simulink model "sfcndemo_stvmgain"  (Simulink 7.6)
settings: Solver=FixedStepDiscrete  SolverMode=SingleTasking  StartTime=0.0  StopTime=4.0  FixedStep=.01  RelTol=1e-3
Description:
  | Time-Varying Matrix Gain C-MEX S-function
settings Model: Creator=The MathWorks Inc.  ExtModeTrigMode=oneshot  ExtModeArmWhenConnect=off  ExtModeAutoUpdateStatusClock=off
settings DataIOCC: LimitDataPoints=off  SaveState=on
settings OptimizationCC: BlockReduction=off  BooleanDataType=off  InitFltsAndDblsToZero=on
settings DebuggingCC: SaveWithParameterizedLinksMsg=none  SignalResolutionControl=TryResolveAllWithWarning  SolverPrmCheckMsg=none  MultiTaskDSMMsg=warning  MultiTaskCondExecSysMsg=none
settings HardwareCC: TargetUnknown=on
settings RTWCC: IncludeERTFirstTime=on
settings CodeAppCC: CustomSymbolStrFcn=$F$N$M
settings GRTTargetCC: TargetFcnLib=ansi_tfl_tmw.mat

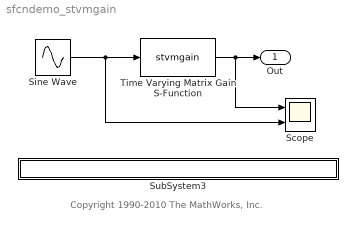
== system sfcndemo_stvmgain ==
  note: Copyright 1990-2010 The MathWorks, Inc.
  Scope : Scope  NumInputPorts=2
      settings: TimeRange=4  YMin=0~-10  YMax=200~10
  Sine Wave : Sin  Amplitude=[1:10 ]  SampleTime=0
  SubSystem3 : Subsystem  mask{filename=stvmgain.c}
      mask init:
      | x=sfundemo_maskdisp;
      settings: AttributesFormatString=\n  OpenFcn=sfundemo_openfcn
      mask Display: disp(x);
  Time Varying Matrix Gain S-Function : S-Function  FunctionName=stvmgain  Parameters=vec, ts  EnableBusSupport=off  mask(S-function: stvmgain){vec=[1.0 1.25 1.5 1.75 2.0], ts=0.1}
      mask prompts: vec "Input vector:"; ts "Sample Time:"
      mask help: This is a S-function block which calculates time- varying matrix gain function.
  Out : Outport  InitialOutput=0
  wires:
  Time Varying Matrix Gain S-Function/1 -> Out/1, Scope/1
  Sine Wave/1 -> Time Varying Matrix Gain S-Function/1, Scope/2

== system sfcndemo_stvmgain/SubSystem3 ==
